simulink model "sigma_delta_4order_CIFF"  (R2024b)
settings: Solver=VariableStepAuto  StartTime=0.0  StopTime=(Mpoints+10)*ts  RelTol=1e-3
InitFcn:
  | fs=256e3;
  | ts=1/fs;
  | osr=128;
  | N=31;
  | Mpoints=2^18;
  | fin=fs*N/Mpoints;
  | a=[6 6 4 2];
  | b=[1 0 0 0 1];
  | c=[1/6 1/4 1/4 1/6];
undefined symbols (not defined in the file): argo, dspblkCoreblockFVToolHelper, gcbh
libraries: SDtoolbox x2
settings Model: Creator=gh  LastModifiedBy=gh

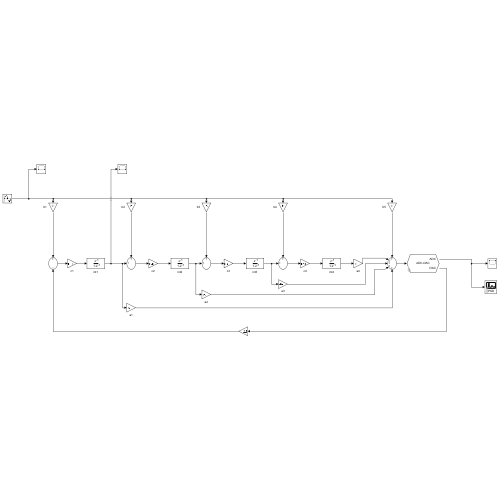
[thumbnail: Simulink's stored preview of the top-level diagram]
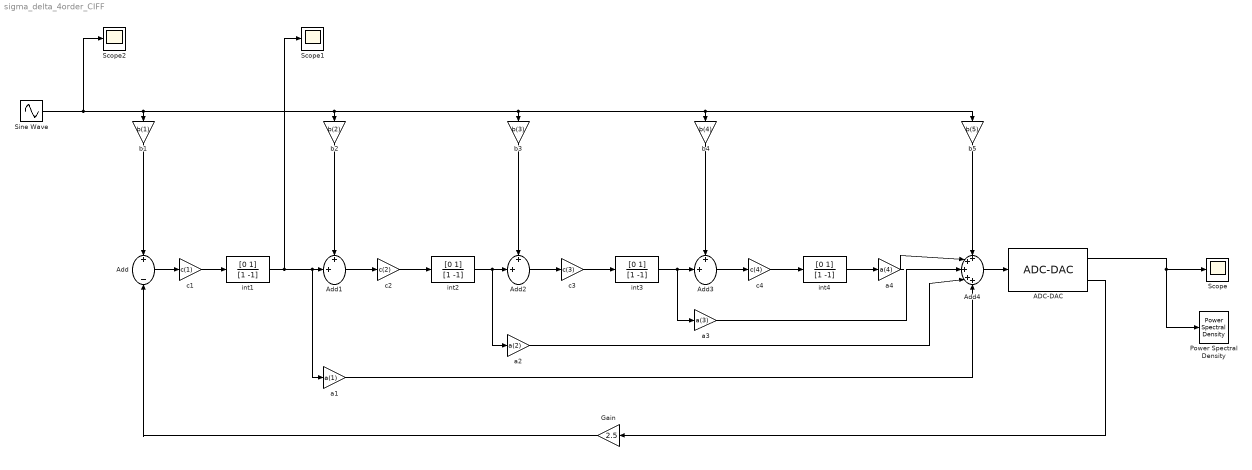
== system sigma_delta_4order_CIFF ==
  ADC-DAC : SDtoolbox/ADC-DAC  k=15  MM=off  match=0  CST=0  VVG=off  argo=argo(:,3)  LF=on  NF=retA.log
      settings: SourceProductName=SDtoolbox
  Add : Sum  Inputs=+-
  Add1 : Sum  Inputs=++|
  Add2 : Sum  Inputs=++|
  Add3 : Sum  Inputs=++|
  Add4 : Sum  Inputs=+++++
  Gain : Gain  Gain=2.5
  Power Spectral Density : SDtoolbox/Power Spectral Density  SN=2  Fs=fs  fBL=0  fBH=fs/(2*osr)  Fin=fin  N=Mpoints  Ntransient=10  VW=off  savename=savemat  Scale_type=logarithmic
      settings: SourceProductName=SDtoolbox
  Scope : Scope
  Scope1 : Scope
  Scope2 : Scope
  Sine Wave : Sin  Amplitude=1.25  Frequency=fin*2*pi  SampleTime=ts
  a1 : Gain  Gain=a(1)
  a2 : Gain  Gain=a(2)
  a3 : Gain  Gain=a(3)
  a4 : Gain  Gain=a(4)
  b1 : Gain  Gain=b(1)
  b2 : Gain  Gain=b(2)
  b3 : Gain  Gain=b(3)
  b4 : Gain  Gain=b(4)
  b5 : Gain  Gain=b(5)
  c1 : Gain  Gain=c(1)
  c2 : Gain  Gain=c(2)
  c3 : Gain  Gain=c(3)
  c4 : Gain  Gain=c(4)
  int{1..4} (4 alike) : DiscreteFilter  LoadFcn=dspblkCoreblockFVToolHelper(gcbh,'load');  Numerator=[0 1]  Denominator=[1 -1]
      settings: CopyFcn=dspblkCoreblockFVToolHelper(gcbh,'copy');  DeleteFcn=dspblkCoreblockFVToolHelper(gcbh,'close');  ModelCloseFcn=dspblkCoreblockFVToolHelper(gcbh,'close');  PreSaveFcn=dspblkCoreblockFVToolHelper(gcbh,'presave');  PostSaveFcn=dspblkCoreblockFVToolHelper(gcbh,'postsave');  CloseFcn=dspblkCoreblockFVToolHelper(gcbh,'close');
  wires:
  c3/1 -> int3/1
  Add3/1 -> c4/1
  a4/1 -> Add4/2
  Add/1 -> c1/1
  c1/1 -> int1/1
  int1/1 -> Scope1/1, a1/1, Add1/2
  Add1/1 -> c2/1
  c2/1 -> int2/1
  int2/1 -> a2/1, Add2/2
  Add2/1 -> c3/1
  int3/1 -> a3/1, Add3/2
  c4/1 -> int4/1
  int4/1 -> a4/1
  Sine Wave/1 -> Scope2/1, b5/1, b4/1, b3/1, b2/1, b1/1
  b1/1 -> Add/1
  b2/1 -> Add1/1
  b3/1 -> Add2/1
  b4/1 -> Add3/1
  b5/1 -> Add4/1
  a3/1 -> Add4/3
  a2/1 -> Add4/4
  a1/1 -> Add4/5
  Add4/1 -> ADC-DAC/1
  ADC-DAC/1 -> Scope/1, Power Spectral Density/1
  ADC-DAC/2 -> Gain/1
  Gain/1 -> Add/2
